simulink library "Digital_8bit_Library"  (R2016a)
settings: Solver=ode45  StartTime=0.0  StopTime=10.0  RelTol=1e-3
libraries: Digital_8bit_Library x19, simulink_extras x17
settings Model: Creator=ronip  LastModifiedBy=Lara
settings SolverCC: AutoInsertRateTranBlk=on
settings DataIOCC: SaveFormat=Array  SignalLoggingSaveFormat=ModelDataLogs  SaveOutput=off  SignalLogging=off  DSMLogging=off  SaveTime=off
settings OptimizationCC: ExpressionDepthLimit=2147483647  StateBitsets=on  DataBitsets=on  OptimizeModelRefInitCode=on  LifeSpan=1
settings DebuggingCC: UnderspecifiedInitializationDetection=Classic  MergeDetectMultiDrivingBlocksExec=none  SolverPrmCheckMsg=warning  FcnCallInpInsideContextMsg=UseLocalSettings  BusObjectLabelMismatch=error  StateNameClashWarn=warning
settings HardwareCC: ProdBitPerPointer=32  ProdLargestAtomicFloat=None  ProdIntDivRoundTo=Undefined  ProdEndianess=Unspecified  ProdWordSize=32  ProdHWDeviceType=32-bit Generic
settings ModelReferenceCC: PropagateSignalLabelsOutOfModel=off
settings RTWCC: SystemTargetFile=ert.tlc  TemplateMakefile=ert_default_tmf  Description=Real-Time Workshop Embedded Coder  GenerateReport=on  IncludeHyperlinkInReport=on  LaunchReport=on  CreateSILPILBlock=SIL  GenerateTraceInfo=on  GenerateTraceReport=on  GenerateTraceReportSl=on  GenerateTraceReportSf=on  GenerateTraceReportEml=on
settings CodeAppCC: IgnoreCustomStorageClasses=off  CustomSymbolStrType=$N$R$M  InternalIdentifier=Classic
settings ERTTargetCC: GenerateSampleERTMain=on  IncludeMdlTerminateFcn=off  ERTCustomFileTemplate=example_file_process.tlc  ConvertIfToSwitch=off  SuppressUnreachableDefaultCases=off
settings ConfigComp: CovModelRefEnable=Off

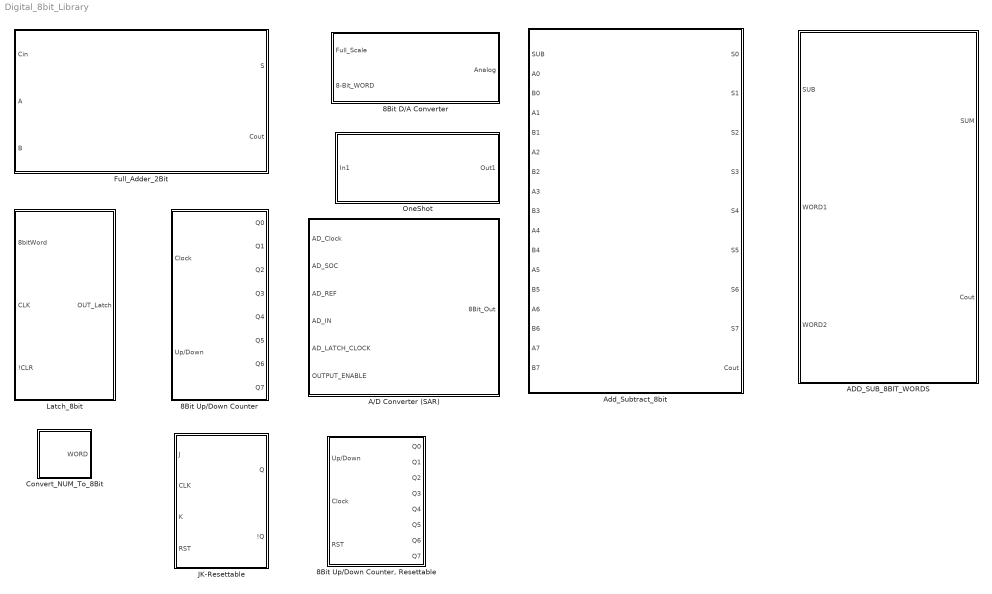
== system Digital_8bit_Library ==
  8Bit D/A Converter : Subsystem
  8Bit Up/Down Counter : Subsystem
  "8Bit Up/Down Counter, Resettable" : Subsystem
  A/D Converter (SAR) : Subsystem
      mask Display: disp('A/D Converter (SAR)')
  ADD_SUB_8BIT_WORDS : Subsystem
  Add_Subtract_8bit : Subsystem
      mask Display:
      | image(imread('AddSub.jpg'))
      | port_label('input',1,'SUB')
      | port_label('input',2,'A0')
      | port_label('input',3,'B0')
      | port_label('input',4,'A1')
      | port_label('input',5,'B1')
      | port_label('input',6,'A2')
      | port_label('input',7,'B2')
      | port_label('input',8,'A3')
      | port_label('input',9,'B3')
      | port_label('input',10,'A4')
      | port_label('input',11,'B4')
      | port_label('input',12,'A5')
      | port_label('input',13,'B5')
      | port_label('input',14,'A6')
      | port_label('input',15,'B6')
      | port_label('input',16,'A7')
      | port_label('input',17,'B7')
      | port_label('output',1,'S0')
      | port_label('output',2,'S1')
      | port_label('output',3,'S2')
      | port_label('output',4,'S3')
      | port_label('output',5,'S4')
      | port_label('output',6,'S5')
      | port_label('output',7,'S6')
      | port_label('output',8,'S7')
      | port_label('output',9,'Cout')
  Convert_NUM_To_8Bit : Subsystem  mask(Convert Decimal number to 8 Bit Representation.){N=8}
      mask prompts: N "Number to convert:"
      mask help:
      | This blocks gets a number from the user, and converts it to an 8Bit
      | representation, Very similar to A/D Converter.
      | Parameters: NUM - The number you wish to convert. (0-255)
      | Output: Boolean 8-Bit vector.
      mask Help:
      | Just enter the number. Remember that the values are represented in 8-Bit format,
      | Therefore the numbers supported are 0-255.\
  Full_Adder_2Bit : Subsystem
      mask Display:
      | image(imread('Full_Adder.jpg'))
      | port_label('input',2,'A')
      | port_label('input',3,'B')
      | port_label('input',1,'Cin')
      | port_label('output',1,'S')
      | port_label('output',2,'Cout')
  JK-Resettable : Subsystem
  Latch_8bit : Subsystem
  OneShot : Subsystem  mask{OneShotTimer=0.001}
      mask prompts: OneShotTimer "Enter One Shot Delay(sec):"
      settings: AttributesFormatString=Delay= %<OneShotTimer>sec
      mask Display: disp('One Shot');

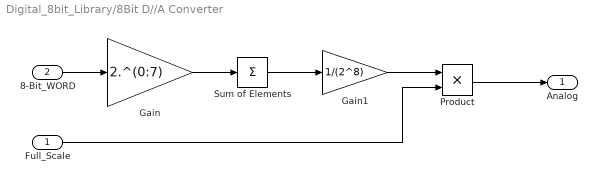
== system Digital_8bit_Library/8Bit D//A Converter ==
  Full_Scale : Inport
  8-Bit_WORD : Inport  Port=2
  Gain : Gain  Gain=2.^(0:7)
  Gain1 : Gain  Gain=1/(2^8)
  Product : Product  RndMeth=Zero
  Sum of Elements : Sum  Inputs=+
  Analog : Outport
  wires:
  Gain/1 -> Sum of Elements/1
  Sum of Elements/1 -> Gain1/1
  Gain1/1 -> Product/1
  Product/1 -> Analog/1
  Full_Scale/1 -> Product/2
  8-Bit_WORD/1 -> Gain/1

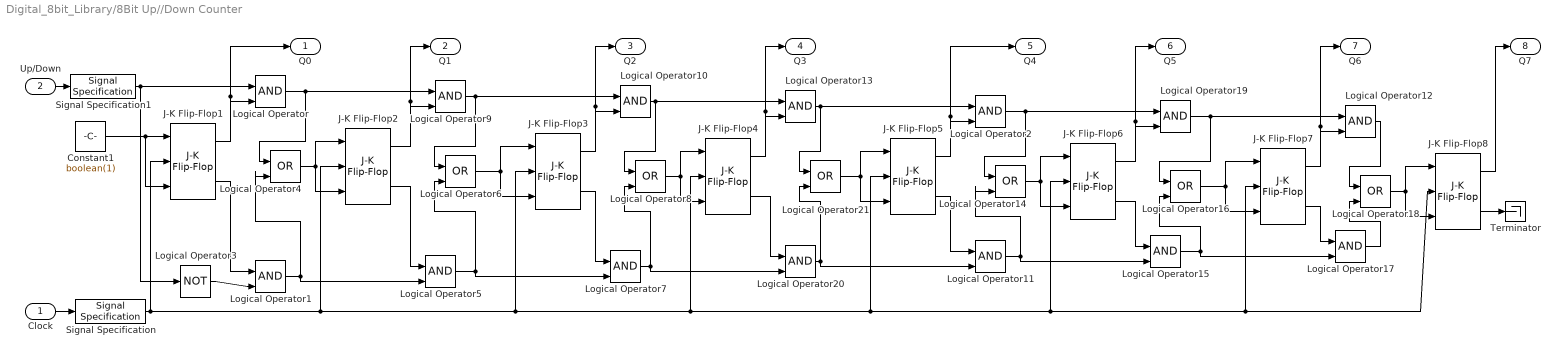
== system Digital_8bit_Library/8Bit Up//Down Counter ==
  Clock : Inport
  Up/Down : Inport  Port=2
  Constant1 : Constant  Value=boolean(1)
  J-K Flip-Flop{1..8} (8 alike) : simulink_extras/Flip Flops/J-K Flip-Flop  SystemSampleTime=-1  initial_condition=0
  Logical Operator{,1..2,5,7,9..13,15,17,19..20} (14 alike) : Logic  IconShape=distinctive  AllPortsSameDT=off  OutDataTypeStr=boolean
  Logical Operator{4,6,8,14,16,18,21} (7 alike) : Logic  Operator=OR  IconShape=distinctive  AllPortsSameDT=off  OutDataTypeStr=boolean
  Logical Operator3 : Logic  Operator=NOT  IconShape=distinctive  AllPortsSameDT=off  OutDataTypeStr=boolean
  Signal Specification : SignalSpecification  OutDataTypeStr=boolean
  Signal Specification1 : SignalSpecification  OutDataTypeStr=boolean
  Terminator : Terminator
  Q0 : Outport  InitialOutput=0
  Q1 : Outport  Port=2  InitialOutput=0
  Q2 : Outport  Port=3  InitialOutput=0
  Q3 : Outport  Port=4  InitialOutput=0
  Q4 : Outport  Port=5  InitialOutput=0
  Q5 : Outport  Port=6  InitialOutput=0
  Q6 : Outport  Port=7  InitialOutput=0
  Q7 : Outport  Port=8  InitialOutput=0
  wires:
  J-K Flip-Flop1/2 -> Logical Operator1/1
  J-K Flip-Flop1/1 -> Q0/1, Logical Operator/2
  Logical Operator/1 -> Logical Operator4/1, Logical Operator9/1
  Clock/1 -> Signal Specification/1
  Constant1/1 -> J-K Flip-Flop1/1, J-K Flip-Flop1/3
  Up/Down/1 -> Signal Specification1/1
  Logical Operator3/1 -> Logical Operator1/2
  Logical Operator1/1 -> Logical Operator4/2, Logical Operator5/2
  J-K Flip-Flop8/2 -> Terminator/1
  J-K Flip-Flop8/1 -> Q7/1
  J-K Flip-Flop2/2 -> Logical Operator5/1
  J-K Flip-Flop4/2 -> Logical Operator20/1
  J-K Flip-Flop3/2 -> Logical Operator7/1
  J-K Flip-Flop3/1 -> Logical Operator10/2, Q2/1
  J-K Flip-Flop4/1 -> Logical Operator13/2, Q3/1
  J-K Flip-Flop2/1 -> Logical Operator9/2, Q1/1
  Logical Operator4/1 -> J-K Flip-Flop2/3, J-K Flip-Flop2/1
  Logical Operator6/1 -> J-K Flip-Flop3/1, J-K Flip-Flop3/3
  Logical Operator5/1 -> Logical Operator6/2, Logical Operator7/2
  Logical Operator7/1 -> Logical Operator8/2, Logical Operator20/2
  Logical Operator8/1 -> J-K Flip-Flop4/1, J-K Flip-Flop4/3
  Logical Operator9/1 -> Logical Operator6/1, Logical Operator10/1
  Logical Operator10/1 -> Logical Operator8/1, Logical Operator13/1
  J-K Flip-Flop6/2 -> Logical Operator15/1
  J-K Flip-Flop5/2 -> Logical Operator11/1
  J-K Flip-Flop5/1 -> Logical Operator2/2, Q4/1
  Logical Operator2/1 -> Logical Operator14/1, Logical Operator19/1
  J-K Flip-Flop7/2 -> Logical Operator17/1
  J-K Flip-Flop7/1 -> Logical Operator12/2, Q6/1
  J-K Flip-Flop6/1 -> Logical Operator19/2, Q5/1
  Logical Operator14/1 -> J-K Flip-Flop6/1, J-K Flip-Flop6/3
  Logical Operator11/1 -> Logical Operator14/2, Logical Operator15/2
  Logical Operator16/1 -> J-K Flip-Flop7/1, J-K Flip-Flop7/3
  Logical Operator15/1 -> Logical Operator16/2, Logical Operator17/2
  Logical Operator17/1 -> Logical Operator18/2
  Logical Operator19/1 -> Logical Operator16/1, Logical Operator12/1
  Logical Operator12/1 -> Logical Operator18/1
  Logical Operator13/1 -> Logical Operator21/1, Logical Operator2/1
  Logical Operator20/1 -> Logical Operator21/2, Logical Operator11/2
  Logical Operator21/1 -> J-K Flip-Flop5/1, J-K Flip-Flop5/3
  Logical Operator18/1 -> J-K Flip-Flop8/1, J-K Flip-Flop8/3
  Signal Specification/1 -> J-K Flip-Flop1/2, J-K Flip-Flop2/2, J-K Flip-Flop8/2, J-K Flip-Flop7/2, J-K Flip-Flop6/2, J-K Flip-Flop5/2, J-K Flip-Flop4/2, J-K Flip-Flop3/2
  Signal Specification1/1 -> Logical Operator3/1, Logical Operator/1

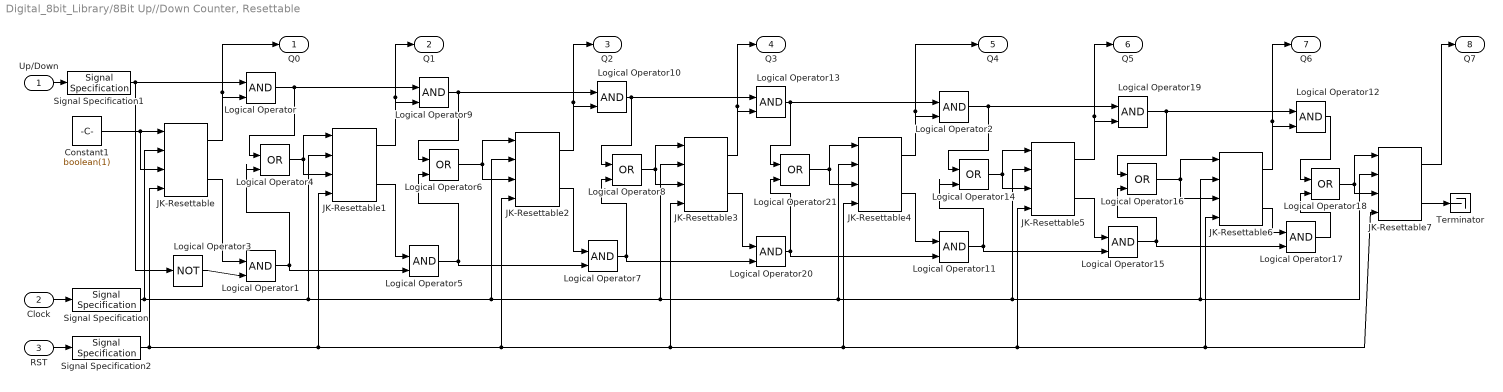
== system Digital_8bit_Library/8Bit Up//Down Counter, Resettable ==
  Up/Down : Inport
  Clock : Inport  Port=2
  RST : Inport  Port=3
  Constant1 : Constant  Value=boolean(1)
  JK-Resettable{,1..7} (8 alike) : Digital_8bit_Library/JK-Resettable  SystemSampleTime=-1
  Logical Operator{,1..2,5,7,9..13,15,17,19..20} (14 alike) : Logic  IconShape=distinctive  AllPortsSameDT=off  OutDataTypeStr=boolean
  Logical Operator{4,6,8,14,16,18,21} (7 alike) : Logic  Operator=OR  IconShape=distinctive  AllPortsSameDT=off  OutDataTypeStr=boolean
  Logical Operator3 : Logic  Operator=NOT  IconShape=distinctive  AllPortsSameDT=off  OutDataTypeStr=boolean
  Signal Specification : SignalSpecification  OutDataTypeStr=boolean
  Signal Specification1 : SignalSpecification  OutDataTypeStr=boolean
  Signal Specification2 : SignalSpecification  OutDataTypeStr=boolean
  Terminator : Terminator
  Q0 : Outport  InitialOutput=0
  Q1 : Outport  Port=2  InitialOutput=0
  Q2 : Outport  Port=3  InitialOutput=0
  Q3 : Outport  Port=4  InitialOutput=0
  Q4 : Outport  Port=5  InitialOutput=0
  Q5 : Outport  Port=6  InitialOutput=0
  Q6 : Outport  Port=7  InitialOutput=0
  Q7 : Outport  Port=8  InitialOutput=0
  wires:
  JK-Resettable/2 -> Logical Operator1/1
  JK-Resettable/1 -> Q0/1, Logical Operator/2
  Logical Operator/1 -> Logical Operator4/1, Logical Operator9/1
  Clock/1 -> Signal Specification/1
  Up/Down/1 -> Signal Specification1/1
  Logical Operator3/1 -> Logical Operator1/2
  Logical Operator1/1 -> Logical Operator4/2, Logical Operator5/2
  JK-Resettable7/2 -> Terminator/1
  JK-Resettable7/1 -> Q7/1
  JK-Resettable1/2 -> Logical Operator5/1
  JK-Resettable3/2 -> Logical Operator20/1
  JK-Resettable2/2 -> Logical Operator7/1
  JK-Resettable2/1 -> Logical Operator10/2, Q2/1
  JK-Resettable3/1 -> Logical Operator13/2, Q3/1
  JK-Resettable1/1 -> Logical Operator9/2, Q1/1
  Logical Operator6/1 -> JK-Resettable2/3, JK-Resettable2/1
  Logical Operator5/1 -> Logical Operator6/2, Logical Operator7/2
  Logical Operator7/1 -> Logical Operator8/2, Logical Operator20/2
  Logical Operator8/1 -> JK-Resettable3/3, JK-Resettable3/1
  Logical Operator9/1 -> Logical Operator6/1, Logical Operator10/1
  Logical Operator10/1 -> Logical Operator8/1, Logical Operator13/1
  JK-Resettable5/2 -> Logical Operator15/1
  JK-Resettable4/2 -> Logical Operator11/1
  JK-Resettable4/1 -> Logical Operator2/2, Q4/1
  Logical Operator2/1 -> Logical Operator14/1, Logical Operator19/1
  JK-Resettable6/2 -> Logical Operator17/1
  JK-Resettable6/1 -> Logical Operator12/2, Q6/1
  JK-Resettable5/1 -> Logical Operator19/2, Q5/1
  Logical Operator14/1 -> JK-Resettable5/3, JK-Resettable5/1
  Logical Operator11/1 -> Logical Operator14/2, Logical Operator15/2
  Logical Operator16/1 -> JK-Resettable6/1, JK-Resettable6/3
  Logical Operator15/1 -> Logical Operator16/2, Logical Operator17/2
  Logical Operator17/1 -> Logical Operator18/2
  Logical Operator19/1 -> Logical Operator16/1, Logical Operator12/1
  Logical Operator12/1 -> Logical Operator18/1
  Logical Operator13/1 -> Logical Operator21/1, Logical Operator2/1
  Logical Operator20/1 -> Logical Operator21/2, Logical Operator11/2
  Logical Operator21/1 -> JK-Resettable4/3, JK-Resettable4/1
  Logical Operator18/1 -> JK-Resettable7/1, JK-Resettable7/3
  Signal Specification/1 -> JK-Resettable6/2, JK-Resettable7/2, JK-Resettable5/2, JK-Resettable4/2, JK-Resettable3/2, JK-Resettable2/2, JK-Resettable1/2, JK-Resettable/2
  Signal Specification1/1 -> Logical Operator3/1, Logical Operator/1
  RST/1 -> Signal Specification2/1
  Signal Specification2/1 -> JK-Resettable/4, JK-Resettable7/4, JK-Resettable6/4, JK-Resettable5/4, JK-Resettable4/4, JK-Resettable3/4, JK-Resettable2/4, JK-Resettable1/4
  Constant1/1 -> JK-Resettable/1, JK-Resettable/3
  Logical Operator4/1 -> JK-Resettable1/1, JK-Resettable1/3

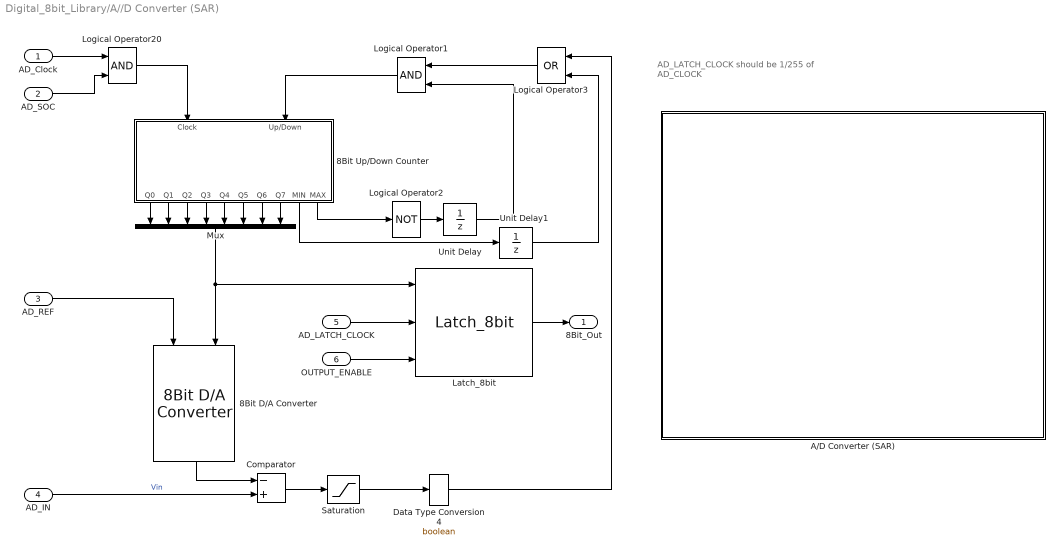
== system Digital_8bit_Library/A//D Converter (SAR) ==
  note: AD_LATCH_CLOCK should
      | be 1/255 of AD_CLOCK
  AD_Clock : Inport
  AD_SOC : Inport  Port=2
  AD_REF : Inport  Port=3
  AD_IN : Inport  Port=4
  AD_LATCH_CLOCK : Inport  Port=5
  OUTPUT_ENABLE : Inport  Port=6
  8Bit D/A Converter : Digital_8bit_Library/8Bit D//A Converter  SystemSampleTime=-1
  8Bit Up/Down Counter : Subsystem  AncestorBlock="Digital_8bit_Library/8Bit Up//Down  Counter"
  A/D Converter (SAR) : Subsystem
      mask init:
      | maskImage= imread('A2D_SAR.jpg');
      mask Display: image(maskImage);
  Comparator : Sum  Inputs=-+  OutDataTypeStr=double
  Data Type Conversion4 : DataTypeConversion  OutDataTypeStr=boolean
  Latch_8bit : Digital_8bit_Library/Latch_8bit  SystemSampleTime=-1
  Logical Operator1 : Logic  IconShape=distinctive  AllPortsSameDT=off  OutDataTypeStr=boolean
  Logical Operator2 : Logic  Operator=NOT  IconShape=distinctive  AllPortsSameDT=off  OutDataTypeStr=boolean
  Logical Operator20 : Logic  IconShape=distinctive  AllPortsSameDT=off  OutDataTypeStr=boolean
  Logical Operator3 : Logic  Operator=OR  IconShape=distinctive  AllPortsSameDT=off  OutDataTypeStr=boolean
  Mux : Mux  Inputs=8
  Saturation : Saturate  UpperLimit=1  LowerLimit=0
  Unit Delay : UnitDelay  InitialCondition=1  SampleTime=-1
  Unit Delay1 : UnitDelay  SampleTime=-1
  8Bit_Out : Outport
  wires:
  8Bit Up/Down Counter/7(Q6) -> Mux/7
  8Bit Up/Down Counter/8(Q7) -> Mux/8
  8Bit Up/Down Counter/1(Q0) -> Mux/1
  8Bit Up/Down Counter/2(Q1) -> Mux/2
  8Bit Up/Down Counter/3(Q2) -> Mux/3
  8Bit Up/Down Counter/4(Q3) -> Mux/4
  8Bit Up/Down Counter/5(Q4) -> Mux/5
  8Bit Up/Down Counter/6(Q5) -> Mux/6
  Mux/1 -> Latch_8bit/1, 8Bit D/A Converter/2
  Comparator/1 -> Saturation/1
  AD_Clock/1 -> Logical Operator20/1
  AD_REF/1 -> 8Bit D/A Converter/1
  8Bit D/A Converter/1 -> Comparator/1
  AD_IN/1 -> Comparator/2  "Vin"
  Saturation/1 -> Data Type Conversion4/1
  OUTPUT_ENABLE/1 -> Latch_8bit/3
  AD_SOC/1 -> Logical Operator20/2
  Logical Operator20/1 -> 8Bit Up/Down Counter/1(Clock)
  Latch_8bit/1 -> 8Bit_Out/1
  AD_LATCH_CLOCK/1 -> Latch_8bit/2
  8Bit Up/Down Counter/10(MAX) -> Logical Operator2/1
  Logical Operator1/1 -> 8Bit Up/Down Counter/2(Up/Down)
  Data Type Conversion4/1 -> Logical Operator3/1
  8Bit Up/Down Counter/9(MIN) -> Unit Delay1/1
  Logical Operator2/1 -> Unit Delay/1
  Logical Operator3/1 -> Logical Operator1/1
  Unit Delay/1 -> Logical Operator1/2
  Unit Delay1/1 -> Logical Operator3/2

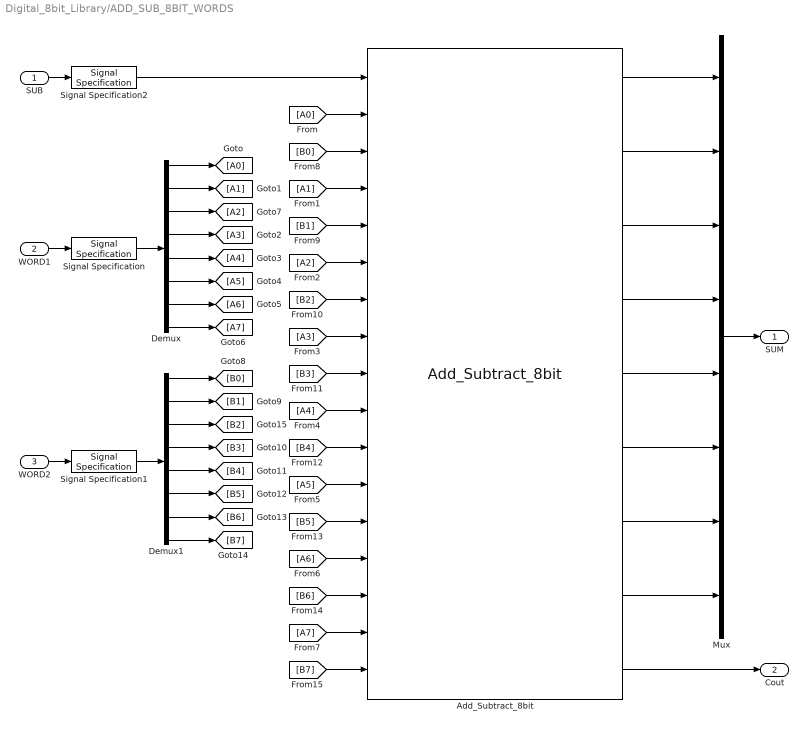
== system Digital_8bit_Library/ADD_SUB_8BIT_WORDS ==
  SUB : Inport
  WORD1 : Inport  Port=2
  WORD2 : Inport  Port=3
  Add_Subtract_8bit : Digital_8bit_Library/Add_Subtract_8bit  SystemSampleTime=-1
  Demux : Demux  Outputs=8
  Demux1 : Demux  Outputs=8
  Mux : Mux  Inputs=8
  Signal Specification : SignalSpecification  OutDataTypeStr=boolean
  Signal Specification1 : SignalSpecification  OutDataTypeStr=boolean
  Signal Specification2 : SignalSpecification  OutDataTypeStr=boolean
  SUM : Outport
  Cout : Outport  Port=2
  wires:
  Add_Subtract_8bit/9 -> Cout/1
  SUB/1 -> Signal Specification2/1
  WORD1/1 -> Signal Specification/1
  Mux/1 -> SUM/1
  WORD2/1 -> Signal Specification1/1
  Add_Subtract_8bit/1 -> Mux/1
  Add_Subtract_8bit/2 -> Mux/2
  Add_Subtract_8bit/3 -> Mux/3
  Add_Subtract_8bit/4 -> Mux/4
  Add_Subtract_8bit/5 -> Mux/5
  Add_Subtract_8bit/6 -> Mux/6
  Add_Subtract_8bit/7 -> Mux/7
  Add_Subtract_8bit/8 -> Mux/8
  Demux/1 -> [A0]
  Demux/2 -> [A1]
  Demux/3 -> [A2]
  Demux/4 -> [A3]
  Demux/5 -> [A4]
  Demux/6 -> [A5]
  Demux/7 -> [A6]
  Demux/8 -> [A7]
  [A0] -> Add_Subtract_8bit/2
  [A1] -> Add_Subtract_8bit/4
  [A2] -> Add_Subtract_8bit/6
  [A3] -> Add_Subtract_8bit/8
  [A4] -> Add_Subtract_8bit/10
  [A5] -> Add_Subtract_8bit/12
  [A6] -> Add_Subtract_8bit/14
  [A7] -> Add_Subtract_8bit/16
  Demux1/1 -> [B0]
  Demux1/2 -> [B1]
  Demux1/3 -> [B2]
  Demux1/4 -> [B3]
  Demux1/5 -> [B4]
  Demux1/6 -> [B5]
  Demux1/7 -> [B6]
  Demux1/8 -> [B7]
  [B0] -> Add_Subtract_8bit/3
  [B1] -> Add_Subtract_8bit/5
  [B2] -> Add_Subtract_8bit/7
  [B3] -> Add_Subtract_8bit/9
  [B4] -> Add_Subtract_8bit/11
  [B5] -> Add_Subtract_8bit/13
  [B6] -> Add_Subtract_8bit/15
  [B7] -> Add_Subtract_8bit/17
  Signal Specification/1 -> Demux/1
  Signal Specification1/1 -> Demux1/1
  Signal Specification2/1 -> Add_Subtract_8bit/1

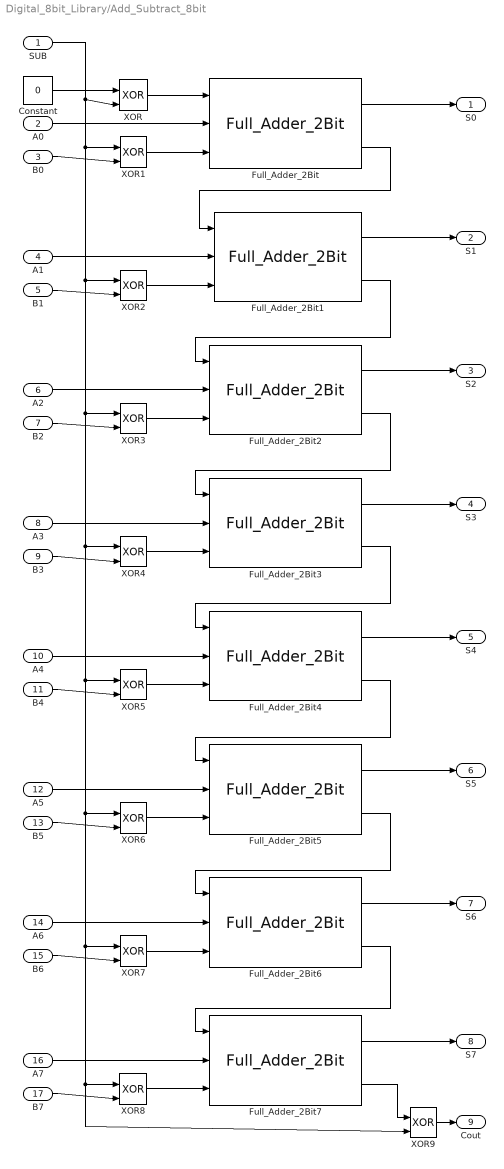
== system Digital_8bit_Library/Add_Subtract_8bit ==
  SUB : Inport
  A0 : Inport  Port=2
  B0 : Inport  Port=3
  A1 : Inport  Port=4
  B1 : Inport  Port=5
  A2 : Inport  Port=6
  B2 : Inport  Port=7
  A3 : Inport  Port=8
  B3 : Inport  Port=9
  A4 : Inport  Port=10
  B4 : Inport  Port=11
  A5 : Inport  Port=12
  B5 : Inport  Port=13
  A6 : Inport  Port=14
  B6 : Inport  Port=15
  A7 : Inport  Port=16
  B7 : Inport  Port=17
  Constant : Constant  Value=0  OutDataTypeStr=boolean
  Full_Adder_2Bit{,1..7} (8 alike) : Digital_8bit_Library/Full_Adder_2Bit  SystemSampleTime=-1
  XOR{,1..9} (10 alike) : Logic  Operator=XOR  IconShape=distinctive  AllPortsSameDT=off  OutDataTypeStr=boolean
  S0 : Outport
  S1 : Outport  Port=2
  S2 : Outport  Port=3
  S3 : Outport  Port=4
  S4 : Outport  Port=5
  S5 : Outport  Port=6
  S6 : Outport  Port=7
  S7 : Outport  Port=8
  Cout : Outport  Port=9
  wires:
  XOR9/1 -> Cout/1
  Full_Adder_2Bit/1 -> S0/1
  Constant/1 -> XOR/1
  SUB/1 -> XOR/2, XOR2/1, XOR3/1, XOR4/1, XOR5/1, XOR7/1, XOR8/1, XOR9/2, XOR6/1, XOR1/1
  B1/1 -> XOR2/2
  Full_Adder_2Bit/2 -> Full_Adder_2Bit1/1
  A1/1 -> Full_Adder_2Bit1/2
  XOR/1 -> Full_Adder_2Bit/1
  A0/1 -> Full_Adder_2Bit/2
  XOR1/1 -> Full_Adder_2Bit/3
  XOR2/1 -> Full_Adder_2Bit1/3
  Full_Adder_2Bit1/1 -> S1/1
  Full_Adder_2Bit2/1 -> S2/1
  Full_Adder_2Bit3/1 -> S3/1
  Full_Adder_2Bit4/1 -> S4/1
  Full_Adder_2Bit5/1 -> S5/1
  Full_Adder_2Bit6/1 -> S6/1
  Full_Adder_2Bit7/1 -> S7/1
  Full_Adder_2Bit1/2 -> Full_Adder_2Bit2/1
  Full_Adder_2Bit2/2 -> Full_Adder_2Bit3/1
  Full_Adder_2Bit3/2 -> Full_Adder_2Bit4/1
  Full_Adder_2Bit4/2 -> Full_Adder_2Bit5/1
  Full_Adder_2Bit5/2 -> Full_Adder_2Bit6/1
  Full_Adder_2Bit6/2 -> Full_Adder_2Bit7/1
  A2/1 -> Full_Adder_2Bit2/2
  XOR3/1 -> Full_Adder_2Bit2/3
  A3/1 -> Full_Adder_2Bit3/2
  XOR4/1 -> Full_Adder_2Bit3/3
  A4/1 -> Full_Adder_2Bit4/2
  XOR5/1 -> Full_Adder_2Bit4/3
  A5/1 -> Full_Adder_2Bit5/2
  XOR6/1 -> Full_Adder_2Bit5/3
  A6/1 -> Full_Adder_2Bit6/2
  XOR7/1 -> Full_Adder_2Bit6/3
  A7/1 -> Full_Adder_2Bit7/2
  XOR8/1 -> Full_Adder_2Bit7/3
  B0/1 -> XOR1/2
  B7/1 -> XOR8/2
  B6/1 -> XOR7/2
  B2/1 -> XOR3/2
  B5/1 -> XOR6/2
  B4/1 -> XOR5/2
  B3/1 -> XOR4/2
  Full_Adder_2Bit7/2 -> XOR9/1

== system Digital_8bit_Library/Convert_NUM_To_8Bit ==
  Constant : Constant  Value=N
  Data Type Conversion : DataTypeConversion  OutDataTypeStr=boolean
  Output 8-bit : MATLAB Function  TreatAsAtomicUnit=on
  WORD : Outport
  wires:
  Constant/1 -> Output 8-bit/1(u)
  Output 8-bit/1(y) -> Data Type Conversion/1
  Data Type Conversion/1 -> WORD/1

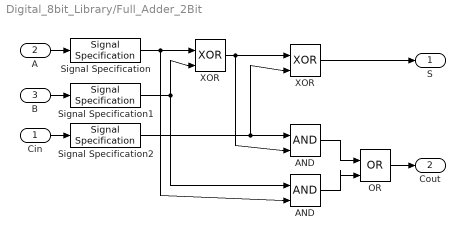
== system Digital_8bit_Library/Full_Adder_2Bit ==
  Cin : Inport
  A : Inport  Port=2
  B : Inport  Port=3
  AND : Logic  IconShape=distinctive  AllPortsSameDT=off  OutDataTypeStr=boolean
  "AND " : Logic  IconShape=distinctive  AllPortsSameDT=off  OutDataTypeStr=boolean
  OR : Logic  Operator=OR  IconShape=distinctive  AllPortsSameDT=off  OutDataTypeStr=boolean
  Signal Specification : SignalSpecification  OutDataTypeStr=boolean
  Signal Specification1 : SignalSpecification  OutDataTypeStr=boolean
  Signal Specification2 : SignalSpecification  OutDataTypeStr=boolean
  XOR : Logic  Operator=XOR  IconShape=distinctive  AllPortsSameDT=off  OutDataTypeStr=boolean
  "XOR " : Logic  Operator=XOR  IconShape=distinctive  AllPortsSameDT=off  OutDataTypeStr=boolean
  S : Outport
  Cout : Outport  Port=2
  wires:
  OR/1 -> Cout/1
  "AND "/1 -> OR/2
  AND/1 -> OR/1
  "XOR "/1 -> S/1
  Cin/1 -> Signal Specification2/1
  XOR/1 -> AND/2, "XOR "/1
  B/1 -> Signal Specification1/1
  A/1 -> Signal Specification/1
  Signal Specification/1 -> "AND "/2, XOR/1
  Signal Specification1/1 -> "AND "/1, XOR/2
  Signal Specification2/1 -> AND/1, "XOR "/2

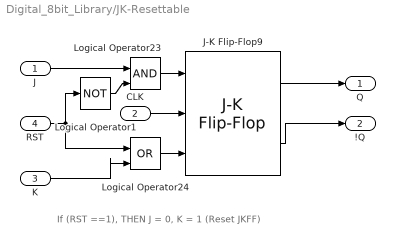
== system Digital_8bit_Library/JK-Resettable ==
  note: If (RST ==1), THEN J = 0, K = 1 (Reset JKFF)
  J : Inport
  CLK : Inport  Port=2
  K : Inport  Port=3
  RST : Inport  Port=4
  J-K Flip-Flop9 : simulink_extras/Flip Flops/J-K Flip-Flop  SystemSampleTime=-1  initial_condition=0
  Logical Operator1 : Logic  Operator=NOT  IconShape=distinctive  AllPortsSameDT=off  OutDataTypeStr=boolean
  Logical Operator23 : Logic  IconShape=distinctive  AllPortsSameDT=off  OutDataTypeStr=boolean
  Logical Operator24 : Logic  Operator=OR  IconShape=distinctive  AllPortsSameDT=off  OutDataTypeStr=boolean
  Q : Outport
  !Q : Outport  Port=2
  wires:
  Logical Operator23/1 -> J-K Flip-Flop9/1
  J/1 -> Logical Operator23/1
  J-K Flip-Flop9/1 -> Q/1
  CLK/1 -> J-K Flip-Flop9/2
  J-K Flip-Flop9/2 -> !Q/1
  RST/1 -> Logical Operator1/1, Logical Operator24/1
  Logical Operator24/1 -> J-K Flip-Flop9/3
  K/1 -> Logical Operator24/2
  Logical Operator1/1 -> Logical Operator23/2

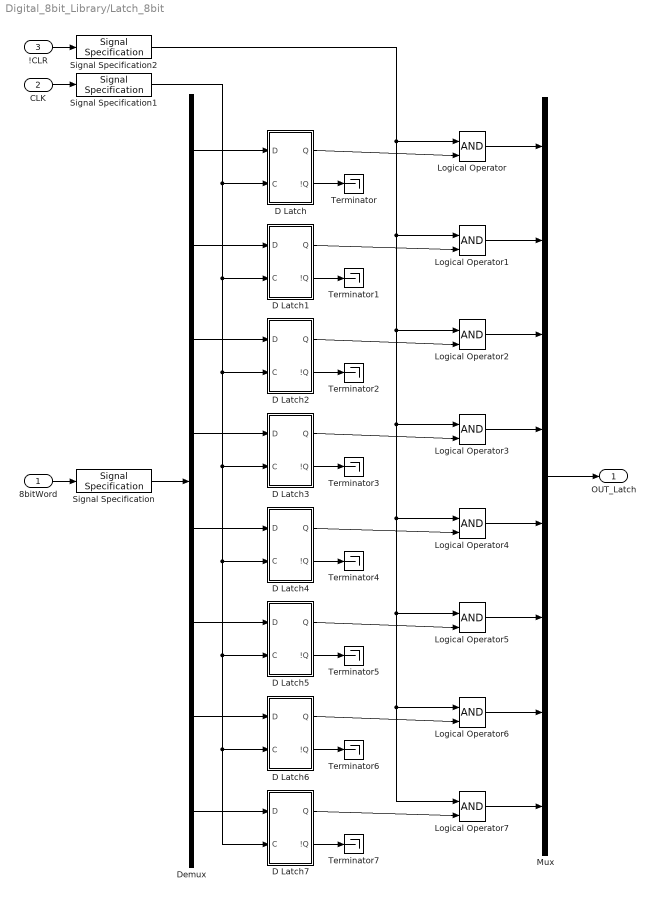
== system Digital_8bit_Library/Latch_8bit ==
  8bitWord : Inport
  CLK : Inport  Port=2
  !CLR : Inport  Port=3
  D Latch : Subsystem  mask(DLatch){}
      mask help: D Latch Flip-Flop Block
      mask Help: web([docroot '/toolbox/simulink/ref_extras/dlatch.html'])
  D Latch1 : Subsystem  mask(DLatch){}
      mask help: D Latch Flip-Flop Block
      mask Help: web([docroot '/toolbox/simulink/ref_extras/dlatch.html'])
  D Latch2 : Subsystem  mask(DLatch){}
      mask help: D Latch Flip-Flop Block
      mask Help: web([docroot '/toolbox/simulink/ref_extras/dlatch.html'])
  D Latch3 : Subsystem  mask(DLatch){}
      mask help: D Latch Flip-Flop Block
      mask Help: web([docroot '/toolbox/simulink/ref_extras/dlatch.html'])
  D Latch4 : Subsystem  mask(DLatch){}
      mask help: D Latch Flip-Flop Block
      mask Help: web([docroot '/toolbox/simulink/ref_extras/dlatch.html'])
  D Latch5 : Subsystem  mask(DLatch){}
      mask help: D Latch Flip-Flop Block
      mask Help: web([docroot '/toolbox/simulink/ref_extras/dlatch.html'])
  D Latch6 : Subsystem  mask(DLatch){}
      mask help: D Latch Flip-Flop Block
      mask Help: web([docroot '/toolbox/simulink/ref_extras/dlatch.html'])
  D Latch7 : Subsystem  mask(DLatch){}
      mask help: D Latch Flip-Flop Block
      mask Help: web([docroot '/toolbox/simulink/ref_extras/dlatch.html'])
  Demux : Demux  Outputs=8
  Logical Operator{,1..7} (8 alike) : Logic  IconShape=distinctive  AllPortsSameDT=off  OutDataTypeStr=boolean
  Mux : Mux  Inputs=8
  Signal Specification : SignalSpecification  OutDataTypeStr=boolean
  Signal Specification1 : SignalSpecification  OutDataTypeStr=boolean
  Signal Specification2 : SignalSpecification  OutDataTypeStr=boolean
  Terminator{,1..7} (8 alike) : Terminator
  OUT_Latch : Outport
  wires:
  Signal Specification2/1 -> Logical Operator/1, Logical Operator5/1, Logical Operator6/1, Logical Operator7/1, Logical Operator4/1, Logical Operator3/1, Logical Operator2/1, Logical Operator1/1
  Signal Specification1/1 -> D Latch/2(C), D Latch1/2(C), D Latch2/2(C), D Latch3/2(C), D Latch4/2(C), D Latch5/2(C), D Latch7/2(C), D Latch6/2(C)
  Signal Specification/1 -> Demux/1
  D Latch/1(Q) -> Logical Operator/2
  Logical Operator7/1 -> Mux/8
  Logical Operator6/1 -> Mux/7
  Logical Operator5/1 -> Mux/6
  Logical Operator4/1 -> Mux/5
  Logical Operator3/1 -> Mux/4
  Logical Operator2/1 -> Mux/3
  Logical Operator1/1 -> Mux/2
  Logical Operator/1 -> Mux/1
  D Latch4/1(Q) -> Logical Operator4/2
  D Latch5/1(Q) -> Logical Operator5/2
  !CLR/1 -> Signal Specification2/1
  Mux/1 -> OUT_Latch/1
  D Latch7/1(Q) -> Logical Operator7/2
  D Latch6/1(Q) -> Logical Operator6/2
  D Latch3/1(Q) -> Logical Operator3/2
  D Latch2/1(Q) -> Logical Operator2/2
  D Latch1/1(Q) -> Logical Operator1/2
  Demux/8 -> D Latch7/1(D)
  Demux/7 -> D Latch6/1(D)
  Demux/6 -> D Latch5/1(D)
  Demux/5 -> D Latch4/1(D)
  Demux/4 -> D Latch3/1(D)
  Demux/3 -> D Latch2/1(D)
  Demux/2 -> D Latch1/1(D)
  Demux/1 -> D Latch/1(D)
  D Latch7/2(!Q) -> Terminator7/1
  D Latch6/2(!Q) -> Terminator6/1
  D Latch5/2(!Q) -> Terminator5/1
  D Latch4/2(!Q) -> Terminator4/1
  D Latch3/2(!Q) -> Terminator3/1
  D Latch2/2(!Q) -> Terminator2/1
  D Latch1/2(!Q) -> Terminator1/1
  D Latch/2(!Q) -> Terminator/1
  CLK/1 -> Signal Specification1/1
  8bitWord/1 -> Signal Specification/1

== system Digital_8bit_Library/OneShot ==
  In1 : Inport
  Clock : Clock
  One-Shot Embedded MATLAB : MATLAB Function  TreatAsAtomicUnit=on
  Out1 : Outport
  wires:
  In1/1 -> One-Shot Embedded MATLAB/1(u)
  One-Shot Embedded MATLAB/1(OC_N_D) -> Out1/1
  Clock/1 -> One-Shot Embedded MATLAB/2(t)

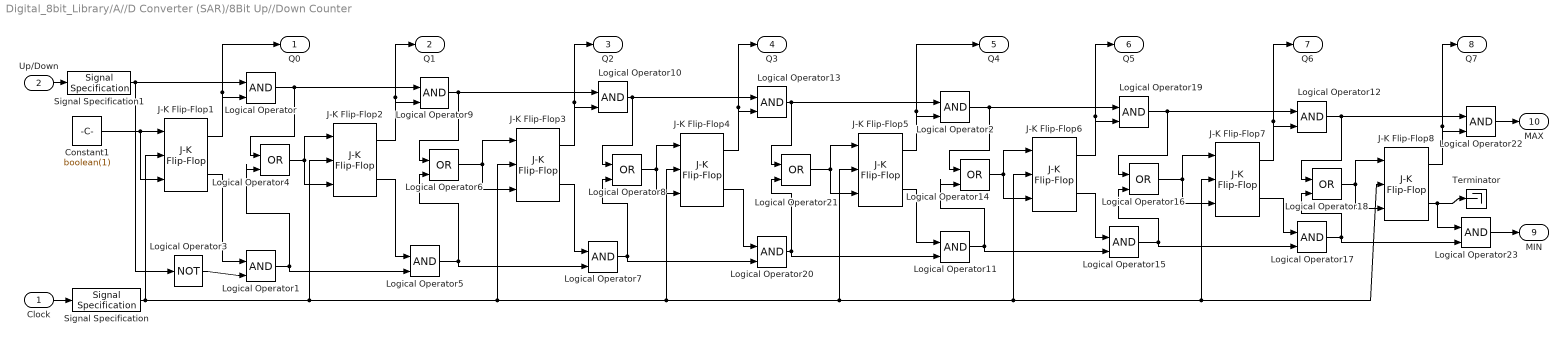
== system Digital_8bit_Library/A//D Converter (SAR)/8Bit Up//Down Counter ==
  Clock : Inport
  Up/Down : Inport  Port=2
  Constant1 : Constant  Value=boolean(1)
  J-K Flip-Flop{1..8} (8 alike) : simulink_extras/Flip Flops/J-K Flip-Flop  SystemSampleTime=-1  initial_condition=0
  Logical Operator{,1..2,5,7,9..13,15,17,19..20,22..23} (16 alike) : Logic  IconShape=distinctive  AllPortsSameDT=off  OutDataTypeStr=boolean
  Logical Operator{4,6,8,14,16,18,21} (7 alike) : Logic  Operator=OR  IconShape=distinctive  AllPortsSameDT=off  OutDataTypeStr=boolean
  Logical Operator3 : Logic  Operator=NOT  IconShape=distinctive  AllPortsSameDT=off  OutDataTypeStr=boolean
  Signal Specification : SignalSpecification  OutDataTypeStr=boolean
  Signal Specification1 : SignalSpecification  OutDataTypeStr=boolean
  Terminator : Terminator
  Q0 : Outport  InitialOutput=0
  Q1 : Outport  Port=2  InitialOutput=0
  Q2 : Outport  Port=3  InitialOutput=0
  Q3 : Outport  Port=4  InitialOutput=0
  Q4 : Outport  Port=5  InitialOutput=0
  Q5 : Outport  Port=6  InitialOutput=0
  Q6 : Outport  Port=7  InitialOutput=0
  Q7 : Outport  Port=8  InitialOutput=0
  MIN : Outport  Port=9  InitialOutput=0
  MAX : Outport  Port=10  InitialOutput=0
  wires:
  Signal Specification1/1 -> Logical Operator/1, Logical Operator3/1
  Signal Specification/1 -> J-K Flip-Flop3/2, J-K Flip-Flop4/2, J-K Flip-Flop5/2, J-K Flip-Flop6/2, J-K Flip-Flop7/2, J-K Flip-Flop8/2, J-K Flip-Flop2/2, J-K Flip-Flop1/2
  Logical Operator18/1 -> J-K Flip-Flop8/3, J-K Flip-Flop8/1
  Logical Operator21/1 -> J-K Flip-Flop5/3, J-K Flip-Flop5/1
  Logical Operator20/1 -> Logical Operator11/2, Logical Operator21/2
  Logical Operator13/1 -> Logical Operator2/1, Logical Operator21/1
  Logical Operator12/1 -> Logical Operator18/1, Logical Operator22/1
  Logical Operator19/1 -> Logical Operator12/1, Logical Operator16/1
  Logical Operator17/1 -> Logical Operator18/2, Logical Operator23/2
  Logical Operator15/1 -> Logical Operator17/2, Logical Operator16/2
  Logical Operator16/1 -> J-K Flip-Flop7/3, J-K Flip-Flop7/1
  Logical Operator11/1 -> Logical Operator15/2, Logical Operator14/2
  Logical Operator14/1 -> J-K Flip-Flop6/3, J-K Flip-Flop6/1
  J-K Flip-Flop6/1 -> Q5/1, Logical Operator19/2
  J-K Flip-Flop7/1 -> Q6/1, Logical Operator12/2
  J-K Flip-Flop7/2 -> Logical Operator17/1
  Logical Operator2/1 -> Logical Operator19/1, Logical Operator14/1
  J-K Flip-Flop5/1 -> Q4/1, Logical Operator2/2
  J-K Flip-Flop5/2 -> Logical Operator11/1
  J-K Flip-Flop6/2 -> Logical Operator15/1
  Logical Operator10/1 -> Logical Operator13/1, Logical Operator8/1
  Logical Operator9/1 -> Logical Operator10/1, Logical Operator6/1
  Logical Operator8/1 -> J-K Flip-Flop4/3, J-K Flip-Flop4/1
  Logical Operator7/1 -> Logical Operator20/2, Logical Operator8/2
  Logical Operator5/1 -> Logical Operator7/2, Logical Operator6/2
  Logical Operator6/1 -> J-K Flip-Flop3/3, J-K Flip-Flop3/1
  Logical Operator4/1 -> J-K Flip-Flop2/1, J-K Flip-Flop2/3
  J-K Flip-Flop2/1 -> Q1/1, Logical Operator9/2
  J-K Flip-Flop4/1 -> Q3/1, Logical Operator13/2
  J-K Flip-Flop3/1 -> Q2/1, Logical Operator10/2
  J-K Flip-Flop3/2 -> Logical Operator7/1
  J-K Flip-Flop4/2 -> Logical Operator20/1
  J-K Flip-Flop2/2 -> Logical Operator5/1
  J-K Flip-Flop8/1 -> Q7/1, Logical Operator22/2
  J-K Flip-Flop8/2 -> Terminator/1, Logical Operator23/1
  Logical Operator1/1 -> Logical Operator5/2, Logical Operator4/2
  Logical Operator3/1 -> Logical Operator1/2
  Up/Down/1 -> Signal Specification1/1
  Constant1/1 -> J-K Flip-Flop1/3, J-K Flip-Flop1/1
  Clock/1 -> Signal Specification/1
  Logical Operator/1 -> Logical Operator9/1, Logical Operator4/1
  J-K Flip-Flop1/1 -> Logical Operator/2, Q0/1
  J-K Flip-Flop1/2 -> Logical Operator1/1
  Logical Operator22/1 -> MAX/1
  Logical Operator23/1 -> MIN/1

== system Digital_8bit_Library/A//D Converter (SAR)/A//D Converter (SAR) ==

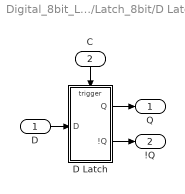
== system Digital_8bit_Library/Latch_8bit/D Latch ==
  D : Inport
  C : Inport  Port=2
  D Latch : Subsystem  TreatAsAtomicUnit=on
  Q : Outport  InitialOutput=0
  !Q : Outport  Port=2  InitialOutput=1
  wires:
  D Latch/2(!Q) -> !Q/1
  D/1 -> D Latch/1(D)
  D Latch/1(Q) -> Q/1
  C/1 -> D Latch/Trigger

== system Digital_8bit_Library/Latch_8bit/D Latch1 ==
  D : Inport
  C : Inport  Port=2
  D Latch : Subsystem  TreatAsAtomicUnit=on
  Q : Outport  InitialOutput=0
  !Q : Outport  Port=2  InitialOutput=1
  wires:
  C/1 -> D Latch/Trigger
  D Latch/1(Q) -> Q/1
  D/1 -> D Latch/1(D)
  D Latch/2(!Q) -> !Q/1

== system Digital_8bit_Library/Latch_8bit/D Latch2 ==
  D : Inport
  C : Inport  Port=2
  D Latch : Subsystem  TreatAsAtomicUnit=on
  Q : Outport  InitialOutput=0
  !Q : Outport  Port=2  InitialOutput=1
  wires:
  D Latch/2(!Q) -> !Q/1
  D/1 -> D Latch/1(D)
  D Latch/1(Q) -> Q/1
  C/1 -> D Latch/Trigger

== system Digital_8bit_Library/Latch_8bit/D Latch3 ==
  D : Inport
  C : Inport  Port=2
  D Latch : Subsystem  TreatAsAtomicUnit=on
  Q : Outport  InitialOutput=0
  !Q : Outport  Port=2  InitialOutput=1
  wires:
  C/1 -> D Latch/Trigger
  D Latch/1(Q) -> Q/1
  D/1 -> D Latch/1(D)
  D Latch/2(!Q) -> !Q/1

== system Digital_8bit_Library/Latch_8bit/D Latch4 ==
  D : Inport
  C : Inport  Port=2
  D Latch : Subsystem  TreatAsAtomicUnit=on
  Q : Outport  InitialOutput=0
  !Q : Outport  Port=2  InitialOutput=1
  wires:
  D Latch/2(!Q) -> !Q/1
  D/1 -> D Latch/1(D)
  D Latch/1(Q) -> Q/1
  C/1 -> D Latch/Trigger

== system Digital_8bit_Library/Latch_8bit/D Latch5 ==
  D : Inport
  C : Inport  Port=2
  D Latch : Subsystem  TreatAsAtomicUnit=on
  Q : Outport  InitialOutput=0
  !Q : Outport  Port=2  InitialOutput=1
  wires:
  C/1 -> D Latch/Trigger
  D Latch/1(Q) -> Q/1
  D/1 -> D Latch/1(D)
  D Latch/2(!Q) -> !Q/1

== system Digital_8bit_Library/Latch_8bit/D Latch6 ==
  D : Inport
  C : Inport  Port=2
  D Latch : Subsystem  TreatAsAtomicUnit=on
  Q : Outport  InitialOutput=0
  !Q : Outport  Port=2  InitialOutput=1
  wires:
  D Latch/2(!Q) -> !Q/1
  D/1 -> D Latch/1(D)
  D Latch/1(Q) -> Q/1
  C/1 -> D Latch/Trigger

== system Digital_8bit_Library/Latch_8bit/D Latch7 ==
  D : Inport
  C : Inport  Port=2
  D Latch : Subsystem  TreatAsAtomicUnit=on
  Q : Outport  InitialOutput=0
  !Q : Outport  Port=2  InitialOutput=1
  wires:
  C/1 -> D Latch/Trigger
  D Latch/1(Q) -> Q/1
  D/1 -> D Latch/1(D)
  D Latch/2(!Q) -> !Q/1

== system Digital_8bit_Library/Latch_8bit/D Latch/D Latch ==
  D : Inport
  Trigger : TriggerPort  VariantControl=Variant
  Logic : Logic  Operator=NOT  Inputs=1
  Q : Outport  InitialOutput=0
  !Q : Outport  Port=2  InitialOutput=1
  wires:
  D/1 -> Logic/1, Q/1
  Logic/1 -> !Q/1

== system Digital_8bit_Library/Latch_8bit/D Latch1/D Latch ==
  D : Inport
  Trigger : TriggerPort  VariantControl=Variant
  Logic : Logic  Operator=NOT  Inputs=1
  Q : Outport  InitialOutput=0
  !Q : Outport  Port=2  InitialOutput=1
  wires:
  Logic/1 -> !Q/1
  D/1 -> Q/1, Logic/1

== system Digital_8bit_Library/Latch_8bit/D Latch2/D Latch ==
  D : Inport
  Trigger : TriggerPort  VariantControl=Variant
  Logic : Logic  Operator=NOT  Inputs=1
  Q : Outport  InitialOutput=0
  !Q : Outport  Port=2  InitialOutput=1
  wires:
  D/1 -> Logic/1, Q/1
  Logic/1 -> !Q/1

== system Digital_8bit_Library/Latch_8bit/D Latch3/D Latch ==
  D : Inport
  Trigger : TriggerPort  VariantControl=Variant
  Logic : Logic  Operator=NOT  Inputs=1
  Q : Outport  InitialOutput=0
  !Q : Outport  Port=2  InitialOutput=1
  wires:
  Logic/1 -> !Q/1
  D/1 -> Q/1, Logic/1

== system Digital_8bit_Library/Latch_8bit/D Latch4/D Latch ==
  D : Inport
  Trigger : TriggerPort  VariantControl=Variant
  Logic : Logic  Operator=NOT  Inputs=1
  Q : Outport  InitialOutput=0
  !Q : Outport  Port=2  InitialOutput=1
  wires:
  D/1 -> Logic/1, Q/1
  Logic/1 -> !Q/1

== system Digital_8bit_Library/Latch_8bit/D Latch5/D Latch ==
  D : Inport
  Trigger : TriggerPort  VariantControl=Variant
  Logic : Logic  Operator=NOT  Inputs=1
  Q : Outport  InitialOutput=0
  !Q : Outport  Port=2  InitialOutput=1
  wires:
  Logic/1 -> !Q/1
  D/1 -> Q/1, Logic/1

== system Digital_8bit_Library/Latch_8bit/D Latch6/D Latch ==
  D : Inport
  Trigger : TriggerPort  VariantControl=Variant
  Logic : Logic  Operator=NOT  Inputs=1
  Q : Outport  InitialOutput=0
  !Q : Outport  Port=2  InitialOutput=1
  wires:
  D/1 -> Logic/1, Q/1
  Logic/1 -> !Q/1

== system Digital_8bit_Library/Latch_8bit/D Latch7/D Latch ==
  D : Inport
  Trigger : TriggerPort  VariantControl=Variant
  Logic : Logic  Operator=NOT  Inputs=1
  Q : Outport  InitialOutput=0
  !Q : Outport  Port=2  InitialOutput=1
  wires:
  Logic/1 -> !Q/1
  D/1 -> Q/1, Logic/1

== matlab function Digital_8bit_Library/Convert_NUM_To_8Bit/Output 8-bit ==
  data: u input; y output
function y = fcn(u)
%#eml
tmp = u;
y = zeros(8,1);
for i=8:-1:1
    if (tmp >= 2^(i-1))
        y(i) = 1;
        tmp = tmp - 2^(i-1);
    else
        y(i) = 0;
    end
end

== matlab function Digital_8bit_Library/OneShot/One-Shot Embedded MATLAB ==
  data: u input; OC_N_D output; t input; OneShotTimer parameter
function OC_N_D = fcn(u, t, OneShotTimer)
%#eml
% This function implemenOneShotTimer a One-Shot device:
% If the input is '0' for a short duration, the output will remain 
% '0' for a longer duration.
% Parameters:
%   u - the input voltage. '0' := 0-2 volOneShotTimer, '1' := 2-5 volOneShotTimer.
%   t - the simulation time.
%   OneShotTimer - timeduration the One-Shot is set.

persistent counter;
if isempty(counter)
    counter = -1;           % Initial value: OneShot isn't active.
end

% One-Shot needs to be operated, input is '0':
if (u < 2)
    counter = t;    % Move the counter to now.
end

if (t - counter < OneShotTimer)    % Is One-Shot still in place:
    OC_N_D = 0;
else
    OC_N_D = u;
    counter = -1;       % Turn off the OneShot.
end
